simulink model "sim1"  (R2019b)
settings: Solver=VariableStepAuto  StartTime=0.0  StopTime=500  RelTol=1e-3
values from neighbouring files (symbols this model uses):
  c = 1.0791e-05    [simi.mat]
  J = 2.8    [simi.mat]
  ke = 0.483958350954    [simi.mat]
  km = 0.415    [simi.mat]
  L = 0.0048    [simi.mat]
  R = 9.65    [simi.mat]
  V = 12    [simi.mat]
libraries: simulink x2
settings Model: Creator=kishore  LastModifiedBy=kishore

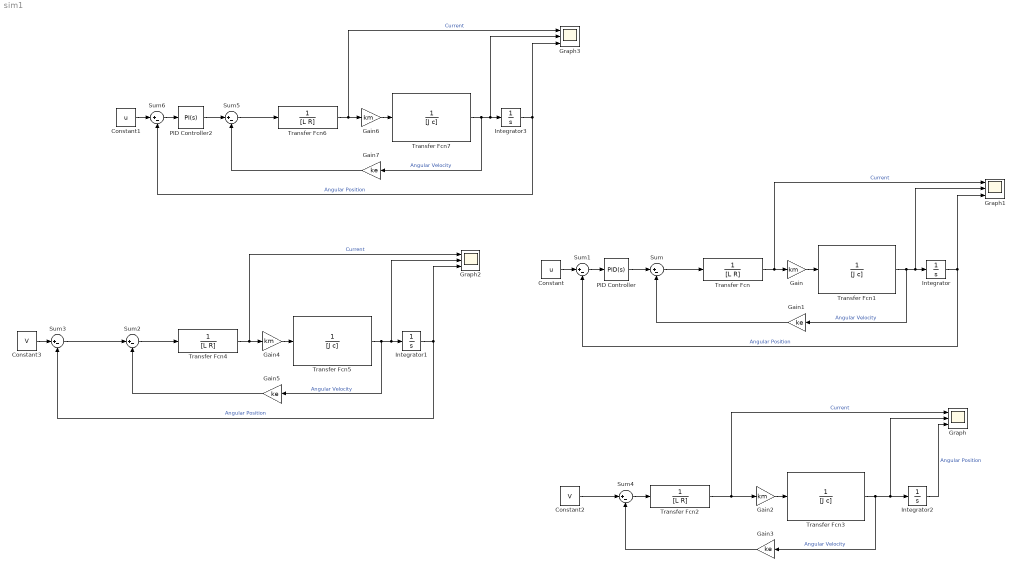
== system sim1 ==
  Constant : Constant  Value=u
  Constant1 : Constant  Value=u
  Constant2 : Constant  Value=V
  Constant3 : Constant  Value=V
  Gain{,2,4,6} (4 alike) : Gain  Gain=km
  Gain{1,3,5,7} (4 alike) : Gain  Gain=ke
  Graph{,1..3} (4 alike) : Scope  NumInputPorts=3
  Integrator{,1..3} (4 alike) : Integrator
  PID Controller : simulink/Continuous/PID Controller  Controller=PID  Form=Parallel  TimeDomain=Continuous-time  SampleTime=-1  IntegratorMethod=Forward Euler  FilterMethod=Forward Euler  ControllerParametersSource=internal  P=0.0432103872000154  I=3.37610838527129e-05  D=4.464906847634274  UseFilter=on  N=11.060836117495227  TunerSelectOption=Transfer Function Based (PID Tuner App)  InitialConditionSource=internal  InitialConditionForIntegrator=0  InitialConditionForFilter=0  DifferentiatorICPrevScaledInput=0  ExternalReset=none  TrackingMode=off  Kt=1  LimitOutput=off  UpperSaturationLimit=inf  LowerSaturationLimit=-inf  LinearizeAsGain=on  AntiWindupMode=none  Kb=1  POutMin=[]  POutMax=[]  IOutMin=[]  IOutMax=[]  DOutMin=[]  DOutMax=[]  NOutMin=[]  NOutMax=[]  SumOutMin=[]  SumOutMax=[]  SaturationOutMin=[]  SaturationOutMax=[]  PParamMin=[]  PParamMax=[]  IParamMin=[]  IParamMax=[]  DParamMin=[]  DParamMax=[]  NParamMin=[]  NParamMax=[]  KbParamMin=[]  KbParamMax=[]  KtParamMin=[]  KtParamMax=[]  KbOutMin=[]  KbOutMax=[]  KtOutMin=[]  KtOutMax=[]  IntegratorOutMin=[]  IntegratorOutMax=[]  FilterOutMin=[]  FilterOutMax=[]  SumI1OutMin=[]  SumI1OutMax=[]  SumI2OutMin=[]  SumI2OutMax=[]  SumI3OutMin=[]  SumI3OutMax=[]  SumI4OutMin=[]  SumI4OutMax=[]  SumDOutMin=[]  SumDOutMax=[]  DifferentiatorOutMin=[]  DifferentiatorOutMax=[]  FilterDiffOutCoefMin=[]  FilterDiffOutCoefMax=[]  ReciprocalOutMin=[]  ReciprocalOutMax=[]  SumDenOutMin=[]  SumDenOutMax=[]  SumNumOutMin=[]  SumNumOutMax=[]  DivideOutMin=[]  DivideOutMax=[]  IntegratorContinuousStateAttributes=''  IntegratorStateMustResolveToSignalObject=off  IntegratorRTWStateStorageClass=Auto  FilterContinuousStateAttributes=''  FilterStateMustResolveToSignalObject=off  FilterRTWStateStorageClass=Auto  ParallelPVariant=InternalParameters  IdealPVariant=Disabled  IVariant=InternalParameters  DVariant=InternalParameters  IntegratorVariant=Continuous  SatVariant=Disabled  AWVariant=Passthrough  PCopyVariant=Disabled  TRVariant=Disabled  FdbkBlocksVariant=Forward  IdealPFdbkVariant=Disabled  SatFdbkVariant=Disabled  DerivativeFilterVariant=ContFilter  NVariant=InternalParameters  NCopyVariant=Disabled  FilterICVariant=InternalICsFilter  IntegratorICVariant=InternalICs  ExternalResetVariant=Disabled  TRSumVariant=Passthrough  SumFdbkVariant=Disabled  SumVariant=Sum_PID
  PID Controller2 : simulink/Continuous/PID Controller  Controller=PI  Form=Parallel  TimeDomain=Continuous-time  SampleTime=-1  IntegratorMethod=Forward Euler  FilterMethod=Forward Euler  ControllerParametersSource=internal  P=1  I=10  D=0  UseFilter=on  N=100  TunerSelectOption=Transfer Function Based (PID Tuner App)  InitialConditionSource=internal  InitialConditionForIntegrator=0  InitialConditionForFilter=0  DifferentiatorICPrevScaledInput=0  ExternalReset=none  TrackingMode=off  Kt=1  LimitOutput=off  UpperSaturationLimit=inf  LowerSaturationLimit=-inf  LinearizeAsGain=on  AntiWindupMode=none  Kb=1  POutMin=[]  POutMax=[]  IOutMin=[]  IOutMax=[]  DOutMin=[]  DOutMax=[]  NOutMin=[]  NOutMax=[]  SumOutMin=[]  SumOutMax=[]  SaturationOutMin=[]  SaturationOutMax=[]  PParamMin=[]  PParamMax=[]  IParamMin=[]  IParamMax=[]  DParamMin=[]  DParamMax=[]  NParamMin=[]  NParamMax=[]  KbParamMin=[]  KbParamMax=[]  KtParamMin=[]  KtParamMax=[]  KbOutMin=[]  KbOutMax=[]  KtOutMin=[]  KtOutMax=[]  IntegratorOutMin=[]  IntegratorOutMax=[]  FilterOutMin=[]  FilterOutMax=[]  SumI1OutMin=[]  SumI1OutMax=[]  SumI2OutMin=[]  SumI2OutMax=[]  SumI3OutMin=[]  SumI3OutMax=[]  SumI4OutMin=[]  SumI4OutMax=[]  SumDOutMin=[]  SumDOutMax=[]  DifferentiatorOutMin=[]  DifferentiatorOutMax=[]  FilterDiffOutCoefMin=[]  FilterDiffOutCoefMax=[]  ReciprocalOutMin=[]  ReciprocalOutMax=[]  SumDenOutMin=[]  SumDenOutMax=[]  SumNumOutMin=[]  SumNumOutMax=[]  DivideOutMin=[]  DivideOutMax=[]  IntegratorContinuousStateAttributes=''  IntegratorStateMustResolveToSignalObject=off  IntegratorRTWStateStorageClass=Auto  FilterContinuousStateAttributes=''  FilterStateMustResolveToSignalObject=off  FilterRTWStateStorageClass=Auto  ParallelPVariant=InternalParameters  IdealPVariant=Disabled  IVariant=InternalParameters  DVariant=Disabled  IntegratorVariant=Continuous  SatVariant=Disabled  AWVariant=Passthrough  PCopyVariant=Disabled  TRVariant=Disabled  FdbkBlocksVariant=Forward  IdealPFdbkVariant=Disabled  SatFdbkVariant=Disabled  DerivativeFilterVariant=Disabled  NVariant=Disabled  NCopyVariant=Disabled_SignalSpec  FilterICVariant=Disabled  IntegratorICVariant=InternalICs  ExternalResetVariant=Disabled  TRSumVariant=Passthrough  SumFdbkVariant=Disabled  SumVariant=Sum_PI
  Sum{,1..6} (7 alike) : Sum  Inputs=|+-
  Transfer Fcn{,2,4,6} (4 alike) : TransferFcn  Denominator=[L R]
  Transfer Fcn{1,3,5,7} (4 alike) : TransferFcn  Denominator=[J c]
  wires:
  Transfer Fcn7/1 -> Graph3/2, Integrator3/1, Gain7/1  "Angular Velocity"
  Transfer Fcn4/1 -> Graph2/1, Gain4/1  "Current"
  Sum3/1 -> Sum2/1
  Transfer Fcn6/1 -> Graph3/1, Gain6/1  "Current"
  Sum5/1 -> Transfer Fcn6/1
  Sum4/1 -> Transfer Fcn2/1
  Sum/1 -> Transfer Fcn/1
  Integrator2/1 -> Graph/3  "Angular Position"
  Gain6/1 -> Transfer Fcn7/1
  Transfer Fcn/1 -> Graph1/1, Gain/1  "Current"
  Sum6/1 -> PID Controller2/1
  Transfer Fcn2/1 -> Graph/1, Gain2/1  "Current"
  Transfer Fcn5/1 -> Graph2/2, Integrator1/1, Gain5/1  "Angular Velocity"
  Gain2/1 -> Transfer Fcn3/1
  Gain5/1 -> Sum2/2
  Constant/1 -> Sum1/1
  Gain7/1 -> Sum5/2
  Integrator3/1 -> Sum6/2, Graph3/3  "Angular Position"
  PID Controller2/1 -> Sum5/1
  Gain4/1 -> Transfer Fcn5/1
  Constant1/1 -> Sum6/1
  Transfer Fcn1/1 -> Graph1/2, Integrator/1, Gain1/1  "Angular Velocity"
  Constant3/1 -> Sum3/1
  Integrator1/1 -> Sum3/2, Graph2/3  "Angular Position"
  Gain/1 -> Transfer Fcn1/1
  Gain1/1 -> Sum/2
  Constant2/1 -> Sum4/1
  PID Controller/1 -> Sum/1
  Sum2/1 -> Transfer Fcn4/1
  Transfer Fcn3/1 -> Graph/2, Integrator2/1, Gain3/1  "Angular Velocity"
  Gain3/1 -> Sum4/2
  Sum1/1 -> PID Controller/1
  Integrator/1 -> Sum1/2, Graph1/3  "Angular Position"
